simulink model "med_sim"  (R2017b)
settings: Solver=ode4  StartTime=0.0  StopTime=100  FixedStep=0.1  RelTol=1e-3
values from neighbouring files (symbols this model uses):
  A = [A11 A12 A13 A14; A21 A22 A23 A24; A31 A32 A33 A34; A41 A42 A43 A44]    [oneforall.m]
  B = [0;0;0;1/jm]    [oneforall.m]
  C = eye(4)    [oneforall.m]
undefined symbols (not defined in the file or in its folder): Kpole
settings Model: Creator=lencs  LastModifiedBy=lencs

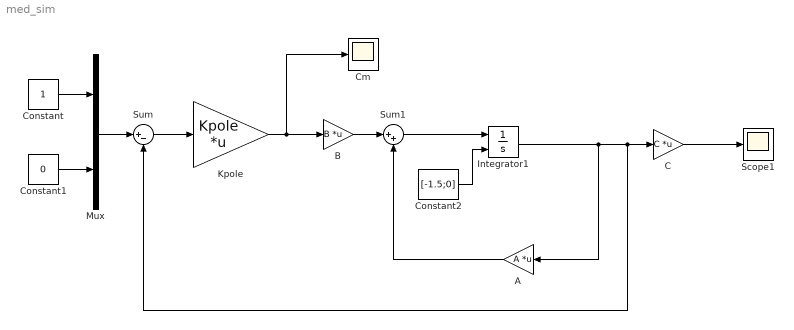
== system med_sim ==
  "A " : Gain  Gain=A  Multiplication=Matrix(K*u)
  B : Gain  Gain=B  Multiplication=Matrix(K*u)
  C : Gain  Gain=C  Multiplication=Matrix(K*u)
  Cm : Scope
  Constant : Constant
  Constant1 : Constant  Value=0
  Constant2 : Constant  Value=[-1.5;0]
  Integrator1 : Integrator  InitialConditionSource=external  InitialCondition=[0.1;0;0;0]
  Kpole : Gain  Gain=Kpole  Multiplication=Matrix(K*u)
  Mux : Mux  Inputs=2
  Scope1 : Scope
  Sum : Sum  Inputs=|+-
  Sum1 : Sum  Inputs=|++
  wires:
  Constant/1 -> Mux/1
  Mux/1 -> Sum/1
  Sum/1 -> Kpole/1
  Sum1/1 -> Integrator1/1
  Integrator1/1 -> Sum/2, C/1, "A "/1
  C/1 -> Scope1/1
  "A "/1 -> Sum1/2
  B/1 -> Sum1/1
  Constant1/1 -> Mux/2
  Constant2/1 -> Integrator1/2
  Kpole/1 -> Cm/1, B/1
